simulink model "suspension_model"  (R2020b)
settings: Solver=ode4  StartTime=0.0  StopTime=T  FixedStep=step  RelTol=1e-3
values from neighbouring files (symbols this model uses):
  b1 = 350    [parameters.m]
  b2 = 15020    [parameters.m]
  k1 = 80000    [parameters.m]
  k2 = 500000    [parameters.m]
  M1 = 2500    [parameters.m]
  M2 = 320    [parameters.m]
settings Model: Creator=kpiekorz  LastModifiedBy=kpiekorz
settings DebuggingCC: AlgebraicLoopMsg=error  ArtificialAlgebraicLoopMsg=error
settings RTWCC: GenCodeOnly=on

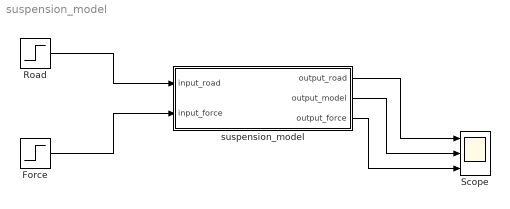
== system suspension_model ==
  Force : Step  Time=0  After=10  SampleTime=0
  Road : Step  Time=0  After=0  SampleTime=0
  Scope : Scope  NumInputPorts=3
  suspension_model : Subsystem
  wires:
  Road/1 -> suspension_model/1(input_road)
  Force/1 -> suspension_model/2(input_force)
  suspension_model/2(output_model) -> Scope/2
  suspension_model/1(output_road) -> Scope/1
  suspension_model/3(output_force) -> Scope/3

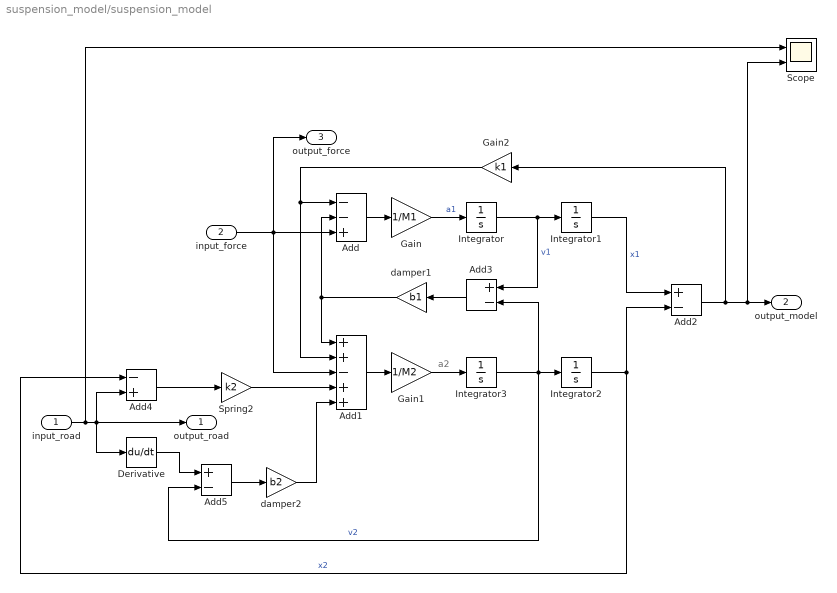
== system suspension_model/suspension_model ==
  note: a2
  input_road : Inport
  input_force : Inport  Port=2
  Add : Sum  Inputs=--+
  Add1 : Sum  Inputs=++-++
  Add2 : Sum  Inputs=+-
  Add3 : Sum  Inputs=+-
  Add4 : Sum  Inputs=-+
  Add5 : Sum  Inputs=+-
  Derivative : Derivative
  Gain : Gain  Gain=1/M1
  Gain1 : Gain  Gain=1/M2
  Gain2 : Gain  Gain=k1
  Integrator{,1..3} (4 alike) : Integrator
  Scope : Scope  NumInputPorts=2
  Spring2 : Gain  Gain=k2
  damper1 : Gain  Gain=b1
  damper2 : Gain  Gain=b2
  output_road : Outport
  output_model : Outport  Port=2
  output_force : Outport  Port=3
  wires:
  Add3/1 -> damper1/1
  damper2/1 -> Add1/5
  Integrator/1 -> Add3/1, Integrator1/1  "v1"
  damper1/1 -> Add/2, Add1/1
  Add1/1 -> Gain1/1
  Integrator1/1 -> Add2/1  "x1"
  Integrator3/1 -> Integrator2/1, Add5/2, Add3/2  "v2"
  Add5/1 -> damper2/1
  Add2/1 -> Scope/2, output_model/1, Gain2/1
  Derivative/1 -> Add5/1
  Add4/1 -> Spring2/1
  Gain/1 -> Integrator/1  "a1"
  Add/1 -> Gain/1
  input_road/1 -> Scope/1, output_road/1, Add4/2, Derivative/1
  Gain2/1 -> Add1/2, Add/1
  input_force/1 -> output_force/1, Add1/3, Add/3
  Integrator2/1 -> Add4/1, Add2/2  "x2"
  Gain1/1 -> Integrator3/1
  Spring2/1 -> Add1/4
